simulink model "model"  (R2023b)
settings: Solver=FixedStepAuto  StartTime=0.0  StopTime=130  FixedStep=0.001  RelTol=1e-3
undefined symbols (not defined in the file): d1, d2, fi0, R, theta1, theta2, theta3, theta4, x0, y0
settings Model: Creator=Damian  LastModifiedBy=Damian

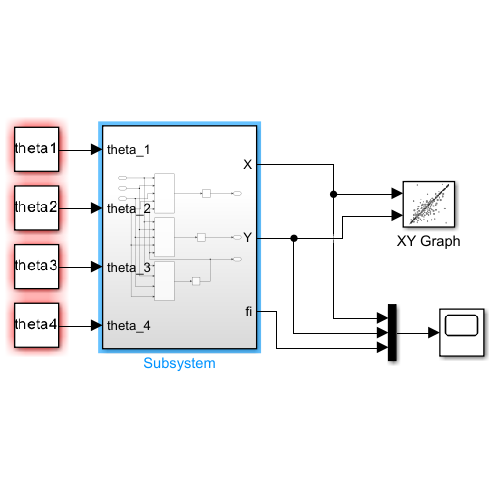
[thumbnail: Simulink's stored preview of the top-level diagram]
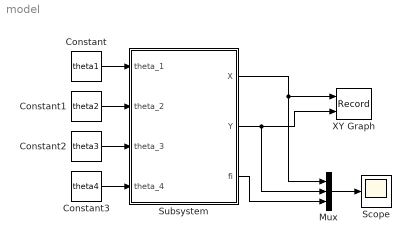
== system model ==
  Constant : Constant  Value=theta1
  Constant1 : Constant  Value=theta2
  Constant2 : Constant  Value=theta3
  Constant3 : Constant  Value=theta4
  Mux : Mux  Inputs=3
  Scope : Scope
  Subsystem : Subsystem
  XY Graph : Record  FileSettingsInternal="{\"entries\":[{\"content\":{\"excelSettings\":{\"content\":{},\"type\":\"Streamout.ExcelSettings\"}},\"type\":\"Streamout.FileSettingStorage\",\"uuid\":\"\"}],\"packageUris\":[\"http:\\/\\/schema.mathworks.com\\/mf0\\/streamout_blocks\\/R2020a\"],\"version\":\"1.0\"}"  Layout=[1 1]  SignalsInternal="{\"entries\":[{\"content\":{\"signals\":[{\"content\":{\"blockPath\":[],\"dimensions\":[1],\"domain\":\"\",\"lineColor\":\"#a2142f\",\"plots\":[ 1 ],\"port\":1,\"sid\":[\"\"],\"signalID\":1,\"signalName\":\"Subsystem:1\"},\"type\":\"RecordBlkView.Signal\",\"uuid\":\"\"},{\"content\":{\"blockPath\":[],\"dimensions\":[1],\"domain\":\"\",\"lineColor\":\"#139fff\",\"plots\":[ 1 ],\"port\":2,\"sid\":[\"\"],\"signalID\":2,\"signalName\":\"Subsystem:2\"},\"type\":\"RecordBlkView.Signal\",\"uuid\":\"\"}]},\"type\":\"RecordBlkView.InputSignals\",\"uuid\":\"\"}],\"packageUris\":[\"http:\\/\\/schema.mathworks.com\\/mf0\\/streamout_blocks\\/R2020a\"],\"version\":\"1.0\"}"  VisualizationBindings="{\"xyplotplugin\":{\"info\":[{\"series\":[{\"bindingParametersList\":[{\"parameter\":\"X-Axis\",\"signalID\":1,\"signalName\":\"Subsystem:1\"},{\"parameter\":\"Y-Axis\",\"signalID\":2,\"signalName\":\"Subsystem:2\"}],\"seriesID\":0}],\"subplotID\":1}]}}"  CompatibilityTag=XY
  wires:
  Subsystem/1(X) -> Mux/1, XY Graph/1
  Subsystem/2(Y) -> Mux/2, XY Graph/2
  Constant/1 -> Subsystem/1(theta_1)
  Constant1/1 -> Subsystem/2(theta_2)
  Constant2/1 -> Subsystem/3(theta_3)
  Constant3/1 -> Subsystem/4(theta_4)
  Subsystem/3(fi) -> Mux/3
  Mux/1 -> Scope/1

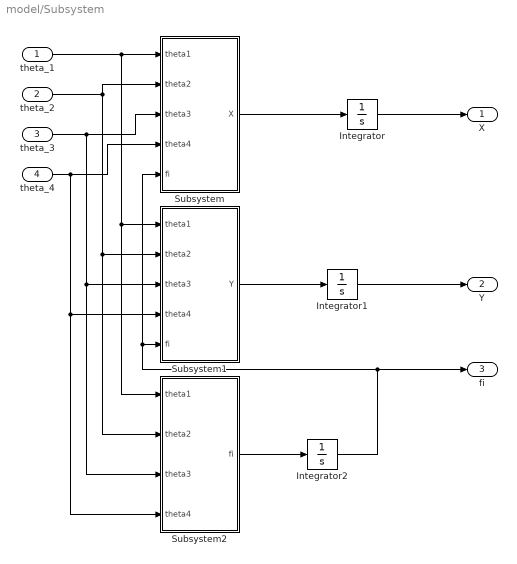
== system model/Subsystem ==
  theta_1 : Inport
  theta_2 : Inport  Port=2
  theta_3 : Inport  Port=3
  theta_4 : Inport  Port=4
  Integrator : Integrator  InitialCondition=x0
  Integrator1 : Integrator  InitialCondition=y0
  Integrator2 : Integrator  InitialCondition=fi0
  Subsystem : Subsystem
  Subsystem1 : Subsystem
  Subsystem2 : Subsystem
  X : Outport
  Y : Outport  Port=2
  fi : Outport  Port=3
  wires:
  theta_1/1 -> Subsystem/1(theta1), Subsystem2/1(theta1), Subsystem1/1(theta1)
  theta_4/1 -> Subsystem2/4(theta4), Subsystem1/4(theta4), Subsystem/4(theta4)
  theta_3/1 -> Subsystem2/3(theta3), Subsystem1/3(theta3), Subsystem/3(theta3)
  theta_2/1 -> Subsystem2/2(theta2), Subsystem1/2(theta2), Subsystem/2(theta2)
  Subsystem/1(X) -> Integrator/1
  Subsystem1/1(Y) -> Integrator1/1
  Integrator/1 -> X/1
  Integrator1/1 -> Y/1
  Subsystem2/1(fi) -> Integrator2/1
  Integrator2/1 -> fi/1, Subsystem/5(fi), Subsystem1/5(fi)

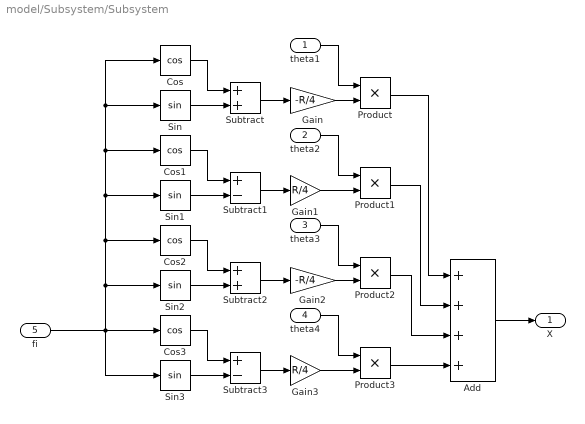
== system model/Subsystem/Subsystem ==
  theta1 : Inport
  theta2 : Inport  Port=2
  theta3 : Inport  Port=3
  theta4 : Inport  Port=4
  fi : Inport  Port=5
  Add : Sum  Inputs=++++
  Cos{,1..3} (4 alike) : Trigonometry  Operator=cos
  Gain : Gain  Gain=-R/4
  Gain1 : Gain  Gain=R/4
  Gain2 : Gain  Gain=-R/4
  Gain3 : Gain  Gain=R/4
  Product{,1..3} (4 alike) : Product
  Sin{,1..3} (4 alike) : Trigonometry
  Subtract : Sum
  Subtract1 : Sum  Inputs=+-
  Subtract2 : Sum
  Subtract3 : Sum  Inputs=+-
  X : Outport
  wires:
  theta2/1 -> Product1/1
  fi/1 -> Sin/1, Cos/1, Cos1/1, Sin1/1, Cos2/1, Sin2/1, Cos3/1, Sin3/1
  Cos/1 -> Subtract/1
  Product/1 -> Add/1
  Sin/1 -> Subtract/2
  Sin1/1 -> Subtract1/2
  Cos1/1 -> Subtract1/1
  Sin2/1 -> Subtract2/2
  Cos2/1 -> Subtract2/1
  Cos3/1 -> Subtract3/1
  Sin3/1 -> Subtract3/2
  Subtract/1 -> Gain/1
  Subtract1/1 -> Gain1/1
  Gain2/1 -> Product2/2
  Subtract2/1 -> Gain2/1
  Gain3/1 -> Product3/2
  Subtract3/1 -> Gain3/1
  theta1/1 -> Product/1
  Gain/1 -> Product/2
  Gain1/1 -> Product1/2
  theta3/1 -> Product2/1
  theta4/1 -> Product3/1
  Product1/1 -> Add/2
  Product2/1 -> Add/3
  Product3/1 -> Add/4
  Add/1 -> X/1

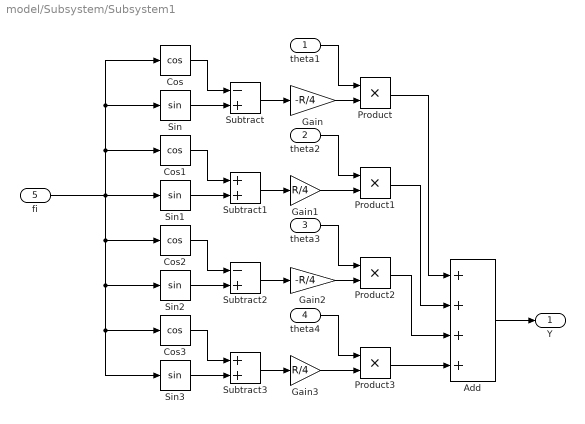
== system model/Subsystem/Subsystem1 ==
  theta1 : Inport
  theta2 : Inport  Port=2
  theta3 : Inport  Port=3
  theta4 : Inport  Port=4
  fi : Inport  Port=5
  Add : Sum  Inputs=++++
  Cos{,1..3} (4 alike) : Trigonometry  Operator=cos
  Gain : Gain  Gain=-R/4
  Gain1 : Gain  Gain=R/4
  Gain2 : Gain  Gain=-R/4
  Gain3 : Gain  Gain=R/4
  Product{,1..3} (4 alike) : Product
  Sin{,1..3} (4 alike) : Trigonometry
  Subtract : Sum  Inputs=-+
  Subtract1 : Sum
  Subtract2 : Sum  Inputs=-+
  Subtract3 : Sum
  Y : Outport
  wires:
  fi/1 -> Cos3/1, Sin3/1, Sin2/1, Cos2/1, Sin/1, Cos/1, Cos1/1, Sin1/1
  Cos/1 -> Subtract/1
  Sin/1 -> Subtract/2
  Cos2/1 -> Subtract2/1
  Cos1/1 -> Subtract1/1
  Sin1/1 -> Subtract1/2
  Sin2/1 -> Subtract2/2
  Cos3/1 -> Subtract3/1
  Sin3/1 -> Subtract3/2
  Subtract/1 -> Gain/1
  Subtract1/1 -> Gain1/1
  Subtract2/1 -> Gain2/1
  Subtract3/1 -> Gain3/1
  theta1/1 -> Product/1
  Gain/1 -> Product/2
  theta2/1 -> Product1/1
  Gain1/1 -> Product1/2
  theta3/1 -> Product2/1
  Gain2/1 -> Product2/2
  theta4/1 -> Product3/1
  Gain3/1 -> Product3/2
  Product/1 -> Add/1
  Product1/1 -> Add/2
  Product2/1 -> Add/3
  Product3/1 -> Add/4
  Add/1 -> Y/1

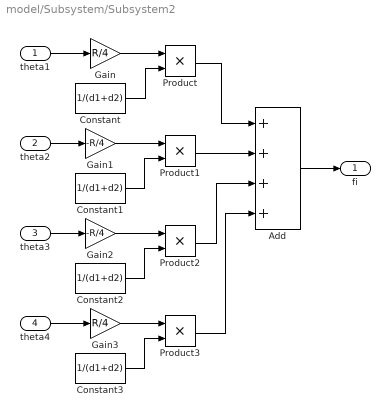
== system model/Subsystem/Subsystem2 ==
  theta1 : Inport
  theta2 : Inport  Port=2
  theta3 : Inport  Port=3
  theta4 : Inport  Port=4
  Add : Sum  Inputs=++++
  Constant{,1..3} (4 alike) : Constant  Value=1/(d1+d2)
  Gain : Gain  Gain=R/4
  Gain1 : Gain  Gain=-R/4
  Gain2 : Gain  Gain=-R/4
  Gain3 : Gain  Gain=R/4
  Product{,1..3} (4 alike) : Product
  fi : Outport
  wires:
  Gain/1 -> Product/1
  theta3/1 -> Gain2/1
  theta1/1 -> Gain/1
  Product3/1 -> Add/4
  Product/1 -> Add/1
  Constant1/1 -> Product1/2
  Gain1/1 -> Product1/1
  theta2/1 -> Gain1/1
  Gain3/1 -> Product3/1
  theta4/1 -> Gain3/1
  Constant/1 -> Product/2
  Gain2/1 -> Product2/1
  Constant2/1 -> Product2/2
  Constant3/1 -> Product3/2
  Product1/1 -> Add/2
  Product2/1 -> Add/3
  Add/1 -> fi/1
